simulink model "fig87_computador_PC"  (R2021a)
settings: Solver=FixedStepAuto  StartTime=0.0  StopTime=tf  FixedStep=Ts  RelTol=1e-3  EnableMultiTasking=on
InitFcn:
  | %leer señal de archivos de Excel
  | %datos = textread('Lampara_CFL.txt');
  |  datos = [
  | 0.E-06	-4.99577E+00	1.52584E-01
  | 1.11E-04	1.87746E+00	1.52584E-01
  | 2.22E-04	8.49173E+00	1.52584E-01
  | 3.33E-04	1.483625E+01	1.52584E-01
  | 4.44E-04	2.192528E+01	1.52584E-01
  | 5.55E-04	2.959697E+01	1.52584E-01
  | 6.66E-04	3.686943E+01	1.52584E-01
  | 7.77E-04	4.391530E+01	1.52584E-01
  | 8.88E-04	5.106907E+01	1.71657E-01
  | 9.99E-04	5.887024E+01	1.71657E-01
  | 1.110E-03	6.697353E+01	1.71657E-01
  | 1.221E-03	7.538973E+01	1.71657E-01
  | 1.332E-03	8.352539E+01	1.90730E-01
  | 1.443E-03	9.111076E+01	1.52584E-01
  | 1.554E-03	9.848033E+01	1.71657E-01
  | 1.665E-03	1.0587148E+02	1.71657E-01
  | 1.776E-03	1.1337053E+02	1.52584E-01
  | 1.887E-03	1.2040561E+02	1.52584E-01
  | 1.998E-03	1.2703067E+02	1.33511E-01
  | 2.109E-03	1.3294359E+02	1.33511E-01
  | 2.220E-03	1.3873782E+02	1.33511E-01
  | 2.331E-03	1.4415440E+02	1.33511E-01
  | 2.442E-03	1.4974362E+02	1.33511E-01
  | 2.553E-03	1.5512783E+02	1.14438E-01
  | 2.664E-03	1.5936830E+02	9.5365E-02
  | 2.775E-03	1.6273478E+02	1.14438E-01
  | 2.886E-03	1.6504384E+02	2.86095E-01
  | 2.997E-03	1.6729895E+02	4.95898E-01
  | 3.108E-03	1.6844269E+02	5.91263E-01
  | 3.219E-03	1.6880955E+02	6.67555E-01
  | 3.330E-03	1.6935984E+02	8.20139E-01
  | 3.441E-03	1.6856138E+02	8.01066E-01
  | 3.552E-03	1.7039568E+02	1.411402E+00
  | 3.663E-03	1.7017988E+02	1.563986E+00
  | 3.774E-03	1.7120493E+02	1.964519E+00
  | 3.885E-03	1.7184154E+02	2.250614E+00
  | 3.996E-03	1.7254289E+02	2.613001E+00
  | 4.107E-03	1.7319029E+02	2.803731E+00
  | 4.218E-03	1.7396717E+02	3.089826E+00
  | 4.329E-03	1.7459299E+02	3.280556E+00
  | 4.440E-03	1.7516486E+02	3.375921E+00
  | 4.551E-03	1.7561804E+02	3.414067E+00
  | 4.662E-03	1.7600648E+02	3.337775E+00
  | 4.773E-03	1.7626544E+02	3.242410E+00
  | 4.884E-03	1.7644887E+02	3.051680E+00
  | 4.995E-03	1.7648124E+02	2.822804E+00
  | 5.106E-03	1.7638413E+02	2.479490E+00
  | 5.217E-03	1.7601727E+02	2.059884E+00
  | 5.328E-03	1.7524039E+02	1.373256E+00
  | 5.439E-03	1.7424771E+02	5.91263E-01
  | 5.550E-03	1.7137757E+02	-9.5365E-02
  | 5.661E-03	1.6563729E+02	-5.7219E-02
  | 5.772E-03	1.5986464E+02	-7.6292E-02
  | 5.883E-03	1.5357407E+02	-7.6292E-02
  | 5.994E-03	1.4727271E+02	-7.6292E-02
  | 6.105E-03	1.4110083E+02	-7.6292E-02
  | 6.216E-03	1.3465920E+02	-9.5365E-02
  | 6.327E-03	1.2822836E+02	-7.6292E-02
  | 6.438E-03	1.2158172E+02	-9.5365E-02
  | 6.549E-03	1.1488113E+02	-7.6292E-02
  | 6.660E-03	1.0815896E+02	-7.6292E-02
  | 6.771E-03	1.0128573E+02	-9.5365E-02
  | 6.882E-03	9.436934E+01	-7.6292E-02
  | 6.993E-03	8.756085E+01	-9.5365E-02
  | 7.104E-03	8.091421E+01	-7.6292E-02
  | 7.215E-03	7.395466E+01	-9.5365E-02
  | 7.326E-03	6.703827E+01	-9.5365E-02
  | 7.437E-03	5.989529E+01	-9.5365E-02
  | 7.548E-03	5.287100E+01	-7.6292E-02
  | 7.659E-03	4.604093E+01	-7.6292E-02
  | 7.770E-03	3.925402E+01	-7.6292E-02
  | 7.881E-03	3.242395E+01	-7.6292E-02
  | 7.992E-03	2.562625E+01	-7.6292E-02
  | 8.103E-03	1.883934E+01	-7.6292E-02
  | 8.214E-03	1.205243E+01	-7.6292E-02
  | 8.325E-03	5.18999E+00	-9.5365E-02
  | 8.436E-03	-1.90983E+00	-7.6292E-02
  | 8.547E-03	-8.56726E+00	-7.6292E-02
  | 8.658E-03	-1.496573E+01	-9.5365E-02
  | 8.769E-03	-2.210871E+01	-9.5365E-02
  | 8.880E-03	-2.972645E+01	-9.5365E-02
  | 8.991E-03	-3.684785E+01	-7.6292E-02
  | 9.102E-03	-4.392609E+01	-7.6292E-02
  | 9.213E-03	-5.110144E+01	-9.5365E-02
  | 9.324E-03	-5.893498E+01	-9.5365E-02
  | 9.435E-03	-6.700590E+01	-9.5365E-02
  | 9.546E-03	-7.534657E+01	-9.5365E-02
  | 9.657E-03	-8.367645E+01	-7.6292E-02
  | 9.768E-03	-9.115392E+01	-7.6292E-02
  | 9.879E-03	-9.852349E+01	-9.5365E-02
  | 9.990E-03	-1.0597938E+02	-9.5365E-02
  | 1.0101E-02	-1.1350001E+02	-7.6292E-02
  | 1.0212E-02	-1.2056746E+02	-7.6292E-02
  | 1.0323E-02	-1.2709541E+02	-5.7219E-02
  | 1.0434E-02	-1.3312702E+02	-5.7219E-02
  | 1.0545E-02	-1.3895362E+02	-3.8146E-02
  | 1.0656E-02	-1.4433783E+02	-5.7219E-02
  | 1.0767E-02	-1.4986231E+02	-5.7219E-02
  | 1.0878E-02	-1.5511704E+02	-3.8146E-02
  | 1.0989E-02	-1.5906618E+02	-1.9073E-02
  | 1.1100E-02	-1.6241108E+02	-1.9073E-02
  | 1.1211E-02	-1.6476330E+02	-2.09803E-01
  | 1.1322E-02	-1.6686735E+02	-3.81460E-01
  | 1.1433E-02	-1.6789240E+02	-4.57752E-01
  | 1.1544E-02	-1.6852901E+02	-5.53117E-01
  | 1.1655E-02	-1.6907930E+02	-6.48482E-01
  | 1.1766E-02	-1.6869086E+02	-6.10336E-01
  | 1.1877E-02	-1.7027699E+02	-1.220672E+00
  | 1.1988E-02	-1.7001803E+02	-1.411402E+00
  | 1.2099E-02	-1.7107545E+02	-1.831008E+00
  | 1.2210E-02	-1.7166890E+02	-2.155249E+00
  | 1.2321E-02	-1.7239183E+02	-2.498563E+00
  | 1.2432E-02	-1.7300686E+02	-2.746512E+00
  | 1.2543E-02	-1.7381611E+02	-3.013534E+00
  | 1.2654E-02	-1.7446351E+02	-3.185191E+00
  | 1.2765E-02	-1.7501380E+02	-3.318702E+00
  | 1.2876E-02	-1.7552093E+02	-3.337775E+00
  | 1.2987E-02	-1.7592016E+02	-3.299629E+00
  | 1.3098E-02	-1.7620070E+02	-3.204264E+00
  | 1.3209E-02	-1.7639492E+02	-3.032607E+00
  | 1.3320E-02	-1.7645966E+02	-2.803731E+00
  | 1.3431E-02	-1.7639492E+02	-2.479490E+00
  | 1.3542E-02	-1.7603885E+02	-2.059884E+00
  | 1.3653E-02	-1.7522960E+02	-1.373256E+00
  | 1.3764E-02	-1.7422613E+02	-5.91263E-01
  | 1.3875E-02	-1.7177680E+02	2.28876E-01
  | 1.3986E-02	-1.6582072E+02	1.71657E-01
  | 1.4097E-02	-1.5967042E+02	1.33511E-01
  | 1.4208E-02	-1.5317484E+02	1.52584E-01
  | 1.4319E-02	-1.4683032E+02	1.52584E-01
  | 1.4430E-02	-1.4069081E+02	1.52584E-01
  | 1.4541E-02	-1.3457288E+02	1.71657E-01
  | 1.4652E-02	-1.2815283E+02	1.52584E-01
  | 1.4763E-02	-1.2159251E+02	1.71657E-01
  | 1.4874E-02	-1.1507535E+02	1.71657E-01
  | 1.4985E-02	-1.0829923E+02	1.71657E-01
  | 1.5096E-02	-1.0137205E+02	1.52584E-01
  | 1.5207E-02	-9.448803E+01	1.52584E-01
  | 1.5318E-02	-8.767954E+01	1.71657E-01
  | 1.5429E-02	-8.102211E+01	1.71657E-01
  | 1.5540E-02	-7.405177E+01	1.71657E-01
  | 1.5651E-02	-6.720012E+01	1.52584E-01
  | 1.5762E-02	-6.013267E+01	1.52584E-01
  | 1.5873E-02	-5.308680E+01	1.52584E-01
  | 1.5984E-02	-4.626752E+01	1.52584E-01
  | 1.6095E-02	-3.950219E+01	1.71657E-01
  | 1.6206E-02	-3.269370E+01	1.71657E-01
  | 1.6317E-02	-2.580968E+01	1.52584E-01
  | 1.6428E-02	-1.893645E+01	1.71657E-01
  | 1.6539E-02	-1.200927E+01	1.33511E-01
  | 1.6650E-02	-4.87708E+00	1.71657E-01
  | 1.6761E-02	2.10405E+00	1.52584E-01
  | 1.6872E-02	8.75069E+00	1.52584E-01
  | 1.6983E-02	1.503047E+01	1.52584E-01
  | 1.7094E-02	2.207634E+01	1.71657E-01
  | 1.7205E-02	2.979119E+01	1.71657E-01
  | 1.7316E-02	3.710681E+01	1.71657E-01
  | 1.7427E-02	4.424979E+01	1.71657E-01
  | 1.7538E-02	5.146830E+01	1.71657E-01
  | 1.7649E-02	5.929105E+01	1.90730E-01
  | 1.7760E-02	6.740513E+01	1.71657E-01
  | 1.7871E-02	7.590765E+01	1.71657E-01
  | 1.7982E-02	8.400015E+01	1.71657E-01
  | 1.8093E-02	9.141288E+01	1.71657E-01
  | 1.8204E-02	9.857744E+01	1.71657E-01
  | 1.8315E-02	1.0589306E+02	1.71657E-01
  | 1.8426E-02	1.1335974E+02	1.52584E-01
  | 1.8537E-02	1.2043798E+02	1.52584E-01
  | 1.8648E-02	1.2691198E+02	1.33511E-01
  | 1.8759E-02	1.3294359E+02	1.33511E-01
  | 1.8870E-02	1.3883493E+02	1.33511E-01
  | 1.8981E-02	1.4431625E+02	1.52584E-01
  | 1.9092E-02	1.4997021E+02	1.33511E-01
  | 1.9203E-02	1.5539758E+02	1.33511E-01
  | 1.9314E-02	1.5941146E+02	9.5365E-02
  | 1.9425E-02	1.6274557E+02	1.14438E-01
  | 1.9536E-02	1.6505463E+02	3.24241E-01
  | 1.9647E-02	1.6727737E+02	4.76825E-01
  | 1.9758E-02	1.6836716E+02	6.10336E-01
  | 1.9869E-02	1.6879876E+02	6.29409E-01
  | 1.9980E-02	1.6938142E+02	8.20139E-01
  | 2.0091E-02	1.6863691E+02	7.62920E-01
  | 2.0202E-02	1.7041726E+02	1.411402E+00
  | 2.0313E-02	1.7022304E+02	1.563986E+00
  | 2.0424E-02	1.7123730E+02	1.964519E+00
  | 2.0535E-02	1.7193865E+02	2.307833E+00
  | 2.0646E-02	1.7260763E+02	2.613001E+00
  | 2.0757E-02	1.7323345E+02	2.860950E+00
  | 2.0868E-02	1.7398875E+02	3.108899E+00
  | 2.0979E-02	1.7460378E+02	3.299629E+00
  | 2.1090E-02	1.7513249E+02	3.375921E+00
  | 2.1201E-02	1.7561804E+02	3.414067E+00
  | 2.1312E-02	1.7598490E+02	3.337775E+00
  | 2.1423E-02	1.7623307E+02	3.223337E+00
  | 2.1534E-02	1.7641650E+02	3.032607E+00
  | 2.1645E-02	1.7647045E+02	2.784658E+00
  | 2.1756E-02	1.7637334E+02	2.460417E+00
  | 2.1867E-02	1.7596332E+02	2.040811E+00
  | 2.1978E-02	1.7521881E+02	1.392329E+00
  | 2.2089E-02	1.7421534E+02	6.10336E-01
  | 2.2200E-02	1.7104308E+02	-9.5365E-02
  | 2.2311E-02	1.6531359E+02	-5.7219E-02
  | 2.2422E-02	1.5942225E+02	-5.7219E-02
  | 2.2533E-02	1.5319642E+02	-5.7219E-02
  | 2.2644E-02	1.4689506E+02	-7.6292E-02
  | 2.2755E-02	1.4071239E+02	-7.6292E-02
  | 2.2866E-02	1.3462683E+02	-7.6292E-02
  | 2.2977E-02	1.2824994E+02	-7.6292E-02
  | 2.3088E-02	1.2168962E+02	-7.6292E-02
  | 2.3199E-02	1.1506456E+02	-7.6292E-02
  | 2.3310E-02	1.0834239E+02	-7.6292E-02
  | 2.3421E-02	1.0141521E+02	-7.6292E-02
  | 2.3532E-02	9.452040E+01	-9.5365E-02
  | 2.3643E-02	8.730189E+01	-7.6292E-02
  | 2.3754E-02	8.063367E+01	-9.5365E-02
  | 2.3865E-02	7.365254E+01	-7.6292E-02
  | 2.3976E-02	6.676852E+01	-7.6292E-02
  | 2.4087E-02	5.974423E+01	-9.5365E-02
  | 2.4198E-02	5.278468E+01	-7.6292E-02
  | 2.4309E-02	4.598698E+01	-9.5365E-02
  | 2.4420E-02	3.923244E+01	-7.6292E-02
  | 2.4531E-02	3.240237E+01	-7.6292E-02
  | 2.4642E-02	2.551835E+01	-9.5365E-02
  | 2.4753E-02	1.866670E+01	-9.5365E-02
  | 2.4864E-02	1.182584E+01	-7.6292E-02
  | 2.4975E-02	4.88787E+00	-9.5365E-02
  | 2.5086E-02	-2.23353E+00	-7.6292E-02
  | 2.5197E-02	-8.88017E+00	-7.6292E-02
  | 2.5308E-02	-1.530022E+01	-7.6292E-02
  | 2.5419E-02	-2.257268E+01	-9.5365E-02
  | 2.5530E-02	-3.019042E+01	-7.6292E-02
  | 2.5641E-02	-3.730103E+01	-7.6292E-02
  | 2.5752E-02	-4.427137E+01	-7.6292E-02
  | 2.5863E-02	-5.136040E+01	-9.5365E-02
  | 2.5974E-02	-5.918315E+01	-9.5365E-02
  | 2.6085E-02	-6.722170E+01	-9.5365E-02
  | 2.6196E-02	-7.561632E+01	-9.5365E-02
  | 2.6307E-02	-8.363329E+01	-7.6292E-02
  | 2.6418E-02	-9.109997E+01	-9.5365E-02
  | 2.6529E-02	-9.842638E+01	-9.5365E-02
  | 2.6640E-02	-1.0591464E+02	-7.6292E-02
  | 2.6751E-02	-1.1350001E+02	-7.6292E-02
  | 2.6862E-02	-1.2059983E+02	-7.6292E-02
  | 2.6973E-02	-1.2710620E+02	-7.6292E-02
  | 2.7084E-02	-1.3338598E+02	-5.7219E-02
  | 2.7195E-02	-1.3916942E+02	-3.8146E-02
  | 2.7306E-02	-1.4452126E+02	-5.7219E-02
  | 2.7417E-02	-1.4999179E+02	-5.7219E-02
  | 2.7528E-02	-1.5519257E+02	-3.8146E-02
  | 2.7639E-02	-1.5914171E+02	-1.9073E-02
  | 2.7750E-02	-1.6245424E+02	-1.9073E-02
  | 2.7861E-02	-1.6474172E+02	-2.09803E-01
  | 2.7972E-02	-1.6678103E+02	-3.81460E-01
  | 2.8083E-02	-1.6784924E+02	-4.76825E-01
  | 2.8194E-02	-1.6852901E+02	-5.53117E-01
  | 2.8305E-02	-1.6911167E+02	-6.67555E-01
  | 2.8416E-02	-1.6866928E+02	-6.10336E-01
  | 2.8527E-02	-1.7032015E+02	-1.220672E+00
  | 2.8638E-02	-1.7005040E+02	-1.392329E+00
  | 2.8749E-02	-1.7111861E+02	-1.792862E+00
  | 2.8860E-02	-1.7167969E+02	-2.155249E+00
  | 2.8971E-02	-1.7244578E+02	-2.460417E+00
  | 2.9082E-02	-1.7305002E+02	-2.708366E+00
  | 2.9193E-02	-1.7385927E+02	-2.975388E+00
  | 2.9304E-02	-1.7448509E+02	-3.166118E+00
  | 2.9415E-02	-1.7504617E+02	-3.280556E+00
  | 2.9526E-02	-1.7553172E+02	-3.318702E+00
  | 2.9637E-02	-1.7592016E+02	-3.280556E+00
  | 2.9748E-02	-1.7622228E+02	-3.185191E+00
  | 2.9859E-02	-1.7641650E+02	-2.994461E+00
  | 2.9970E-02	-1.7649203E+02	-2.765585E+00
  | 3.0081E-02	-1.7643808E+02	-2.460417E+00
  | 3.0192E-02	-1.7610359E+02	-2.002665E+00
  | 3.0303E-02	-1.7527276E+02	-1.335110E+00
  | 3.0414E-02	-1.7429087E+02	-5.34044E-01
  | 3.0525E-02	-1.7194944E+02	1.90730E-01
  | 3.0636E-02	-1.6559413E+02	1.33511E-01
  | 3.0747E-02	-1.5943304E+02	1.52584E-01
  | 3.0858E-02	-1.5294825E+02	1.52584E-01
  | 3.0969E-02	-1.4661452E+02	1.52584E-01
  | 3.1080E-02	-1.4056133E+02	1.52584E-01
  | 3.1191E-02	-1.3452972E+02	1.52584E-01
  | 3.1302E-02	-1.2818520E+02	1.52584E-01
  | 3.1413E-02	-1.2157093E+02	1.52584E-01
  | 3.1524E-02	-1.1488113E+02	1.90730E-01
  | 3.1635E-02	-1.0807264E+02	1.52584E-01
  | 3.1746E-02	-1.0112388E+02	1.71657E-01
  | 3.1857E-02	-9.416433E+01	1.71657E-01
  | 3.1968E-02	-8.731268E+01	1.71657E-01
  | 3.2079E-02	-8.061209E+01	1.71657E-01
  | 3.2190E-02	-7.368491E+01	1.71657E-01
  | 3.2301E-02	-6.689800E+01	1.71657E-01
  | 3.2412E-02	-5.986292E+01	1.71657E-01
  | 3.2523E-02	-5.287100E+01	1.52584E-01
  | 3.2634E-02	-4.601935E+01	1.71657E-01
  | 3.2745E-02	-3.923244E+01	1.52584E-01
  | 3.2856E-02	-3.247790E+01	1.71657E-01
  | 3.2967E-02	-2.561546E+01	1.52584E-01
  | 3.3078E-02	-1.875302E+01	1.71657E-01
  | 3.3189E-02	-1.180426E+01	1.52584E-01
  | ];
  | %generar vectores
  | time = datos(:,1);
  | Va = datos(:,2);
  | Ia = datos(:,3);
  | 
  | %variables (Workspace)
  | Ts=time(2)-time(1);
  | Var_corriente = [time Ia];
  | Var_tension = [time Va];
  | tf = time(end);
libraries: spsACCurrentSourceLib x5, spsSeriesRLCBranchLib x4, spsCurrentMeasurementLib x1, spsVoltageMeasurementLib x1, spsACVoltageSourceLib x1, spspowerguiLib x1
settings Model: NumberOfSteps=5  Creator=aj_us  LastModifiedBy=ajust
settings SolverCC: AlgebraicLoopSolver=TrustRegion
settings DataIOCC: LimitDataPoints=on  ReturnWorkspaceOutputs=off
settings OptimizationCC: LifeSpan=inf
settings DebuggingCC: AllowSymbolicDim=off  SFUnexpectedBacktrackingDiag=warning  SFNoUnconditionalDefaultTransitionDiag=warning  SFExecutionAtInitializationDiag=none  SFMachineParentedDataDiag=warning  ArithmeticOperatorsInVariantConditions=warning
settings ModelReferenceCC: PropagateSignalLabelsOutOfModel=off
settings SFSimCC: SimUseLocalCustomCode=off  CustomCodeUndefinedFunction=UseInterfaceOnly
settings RTWCC: RTWUseLocalCustomCode=off
settings CodeAppCC: StateflowObjectComments=on
settings GRTTargetCC: TargetLangStandard=C89/C90 (ANSI)
settings ConfigComp: CovMetricSettings=dw  CovSaveCumulativeToWorkspaceVar=on  CovSaveSingleToWorkspaceVar=on  CovExternalEMLEnable=off
settings SimscapeCC: SimscapeNormalizeSystem=off

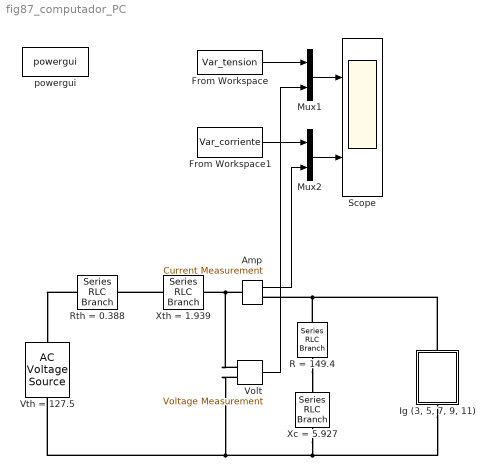
== system fig87_computador_PC ==
  Amp : spsCurrentMeasurementLib/Current Measurement  PhasorSimulation=off  OutputType=Complex  PSBequivalent=0
  From Workspace : FromWorkspace  VariableName=Var_tension  SampleTime=Ts
  From Workspace1 : FromWorkspace  VariableName=Var_corriente  SampleTime=Ts
  "Ig (3, 5, 7, 9, 11)" : Subsystem
      mask Display: plot(-50,-35,50,50-15,[0,9,18,24,29,30,29,24,18,9,0,-9,-18,-24,-29,-30,-29,-24,-18,-9,0],[30,29,24,18,9,0,-9,-18,-24,-29,-30,-29,-24,-18,-9,0,9,18,24,29,30],[-20 5 5 20 5 5],[2 2 12 2 -8 2],[-50 -30],[0 0],[50,30],[0 0],[45 35 40 40 40],[15 15 15 20 10]);
  Mux1 : Mux  Inputs=2
  Mux2 : Mux  Inputs=2
  R = 149.4 : spsSeriesRLCBranchLib/Series RLC Branch  LConnTagsString=__new0  RConnTagsString=__new0  BranchType=R  Resistance=149.4  Inductance=1e-3  SetiL0=off  InitialCurrent=0  Capacitance=1/(2*pi*60*437.9)  Setx0=off  InitialVoltage=0  Measurements=None
  Rth = 0.388 : spsSeriesRLCBranchLib/Series RLC Branch  LConnTagsString=__new0  RConnTagsString=__new0  BranchType=R  Resistance=0.388  Inductance=1e-3  SetiL0=off  InitialCurrent=0  Capacitance=1/(2*pi*60*437.9)  Setx0=off  InitialVoltage=0  Measurements=None
  Scope : Scope  NumInputPorts=2
  Volt : spsVoltageMeasurementLib/Voltage Measurement  PhasorSimulation=off  OutputType=Complex  PSBequivalent=0
  Vth = 127.5 : spsACVoltageSourceLib/AC Voltage Source  Amplitude=sqrt(2)*127.5  Phase=-0.6974  Frequency=60  SampleTime=Ts  Measurements=None  BusType=swing  Pref=10e3  Qref=0  Qmin=-inf  Qmax=+inf
  Xc = 5.927 : spsSeriesRLCBranchLib/Series RLC Branch  LConnTagsString=__new0  RConnTagsString=__new0  BranchType=C  Resistance=758  Inductance=1e-3  SetiL0=off  InitialCurrent=0  Capacitance=1/(2*pi*60*5.927)  Setx0=off  InitialVoltage=0  Measurements=None
  Xth = 1.939 : spsSeriesRLCBranchLib/Series RLC Branch  LConnTagsString=__new0  RConnTagsString=__new0  BranchType=L  Resistance=758  Inductance=1.939/(2*pi*60)  SetiL0=off  InitialCurrent=0  Capacitance=1/(2*pi*60*437.9)  Setx0=off  InitialVoltage=0  Measurements=None
  powergui : spspowerguiLib/powergui  Priority=1  SimulationMode=Discrete  SampleTime=Ts  frequency=60  Iterations=50  frequencyindice=60  Pbase=100e6  ErrMax=1e-4  UnitsV=kV  UnitsW=MW  buscounter=0  FunctionMessages=off  echomessages=off  EnableUseOfTLC=off  CurrentSourceSwitches=off  DisableSnubberDevices=off  DisableRonSwitches=off  DisableVfSwitches=off  DisplayEquations=off  AutomaticDiscreteSolvers=off  SolverType=Tustin/Backward Euler (TBE)  Interpol=off  ExternalGateDelay=off  methode=off  Ts=10  x0status=blocks  SPID=off  SwTol=0  HookPort=off  NonlinearTolerance=1e-4  nMaxIteration=100  ContinueOnMaxIteration=off  RestoreLinks=warning  ResistiveCurrentMeasurement=off  Frange=[0:2:1000]  Ylog=off  Xlog=off  ShowGrid=on  save=on  variable=ZData  structure=ScopeData  ZoomFFT=off  StartTime=1/60  cycles=1  DisplayStyle=2  fundamental=60  FreqAxis=on  MaxFrequency=1200  frequencyindicesteady=1  RmsSteady=2  display=off
  wires:
  From Workspace1/1 -> Mux2/1
  Mux2/1 -> Scope/2
  Amp/1 -> Mux2/2
  Mux1/1 -> Scope/1
  Volt/1 -> Mux1/2
  From Workspace/1 -> Mux1/1
  connections:
  Amp/LConn1 -- Volt/LConn1 -- Xth = 1.939/RConn1
  Rth = 0.388/LConn1 -- Vth = 127.5/RConn1
  Xth = 1.939/LConn1 -- Rth = 0.388/RConn1
  R = 149.4/RConn1 -- Xc = 5.927/LConn1
  R = 149.4/LConn1 -- "Ig (3, 5, 7, 9, 11)"/RConn1 -- Amp/RConn1
  Xc = 5.927/RConn1 -- Volt/LConn2 -- Vth = 127.5/LConn1 -- "Ig (3, 5, 7, 9, 11)"/LConn1

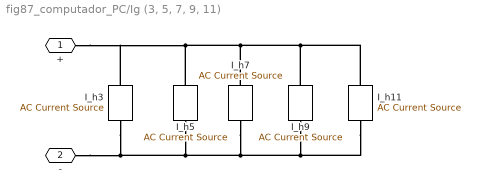
== system fig87_computador_PC/Ig (3, 5, 7, 9, 11) ==
  I_h11 : spsACCurrentSourceLib/AC Current Source  Amplitude=0.09314  Phase=27.21  Frequency=660  SampleTime=Ts  Measurements=None
      settings: SourceProductBaseCode=PS
  I_h3 : spsACCurrentSourceLib/AC Current Source  Amplitude=1.02  Phase=164.8  Frequency=180  SampleTime=Ts  Measurements=None
      settings: SourceProductBaseCode=PS
  I_h5 : spsACCurrentSourceLib/AC Current Source  Amplitude=0.7079  Phase=-30.15  Frequency=300  SampleTime=Ts  Measurements=None
      settings: SourceProductBaseCode=PS
  I_h7 : spsACCurrentSourceLib/AC Current Source  Amplitude=0.3846  Phase=128.4  Frequency=420  SampleTime=Ts  Measurements=None
      settings: SourceProductBaseCode=PS
  I_h9 : spsACCurrentSourceLib/AC Current Source  Amplitude=0.1806  Phase=-91.9  Frequency=540  SampleTime=Ts  Measurements=None
      settings: SourceProductBaseCode=PS
  + : PMIOPort  Side=Left
  - : PMIOPort  Port=2  Side=Right
  connections:
  I_h11/RConn1 -- I_h9/RConn1 -- I_h7/RConn1 -- I_h3/RConn1 -- +/RConn1 -- I_h5/RConn1
  I_h11/LConn1 -- I_h9/LConn1 -- I_h7/LConn1 -- I_h5/LConn1 -- I_h3/LConn1 -- -/RConn1
